simulink model "n99tot96reg55neu_10_8p"  (R2022b)
settings: Solver=VariableStepAuto  StartTime=0.0  StopTime=10.0  RelTol=1e-3
libraries: neural x61
(part 2 of 3)

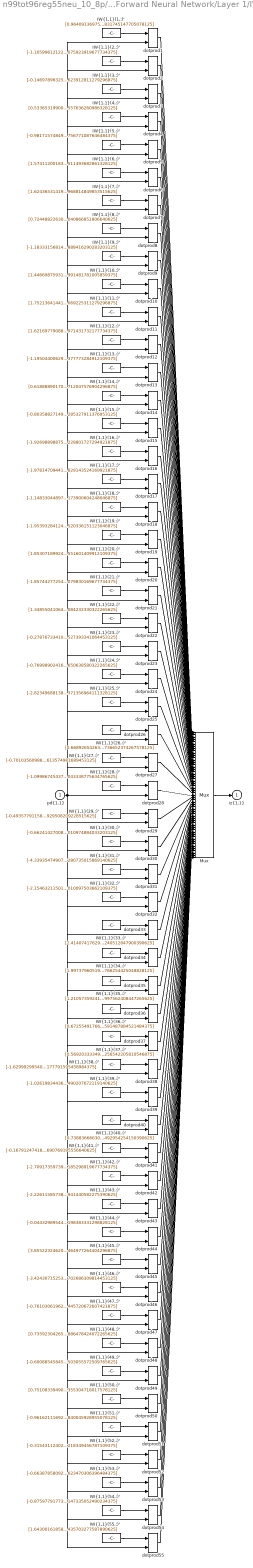
== system n99tot96reg55neu_10_8p/Feed-Forward Neural Network/Layer 1/IW{1,1} ==
  "pd{1,1}" : Inport  PortDimensions=7
      mask Display: e = 0.06;c1 = [120 230 180]/255;c2 = ([120 230 180]+0)/(256+128);c3 = ([120 230 180]+128)/(256+128);patch([0 1 1 0],[0 0 1 1],c1);patch([0 1 1 1-e 1-e 0+e],[0 0 1 1-e 0+e 0+e],c2);patch([0 0 1 1-e 0+e 0+e],[0 1 1 1-e 1-e 0+e],c3);plot([0 1 1 0 0],[0 0 1 1 0]);
  "IW{1,1}(1,:)'" : Constant  Value=[0.96409136975342180075898568247794173657894134521484375;-0.01177306743164707562854243150241018156521022319793701171875;1.5872895079200481927017563066328875720500946044921875;-0.67946510242392033074310120355221442878246307373046875;-1.3804786704522087337210223267902620136737823486328125;0.54905886044986174088222696809680201113224029541015625;0.1319087701998143125070583892011200077831745147705078125]
      mask Display: e = 0.06;c1 = [120 150 230]/255;c2 = ([120 150 230]+0)/383;c3 = ([120 150 230]+128)/383;patch([0 1 1 0],[0 0 1 1],c1);patch([0 1 1 1-e 1-e 0+e],[0 0 1 1-e 0+e 0+e],c2);patch([0 0 1 1-e 0+e 0+e],[0 1 1 1-e 1-e 0+e],c3);plot([0 1 1 0 0],[0 0 1 1 0]);disp('Weights');
  "IW{1,1}(10,:)'" : Constant  Value=[1.44669875931127744905779763939790427684783935546875;1.63028544792287721776347098057158291339874267578125;-0.402402933929877304475297705721459351480007171630859375;-1.5160626699661390315299058784148655831813812255859375;-0.59991510336130193792314457823522388935089111328125;4.485717304041894948340996052138507366180419921875;3.753049417834217305056654367945156991481781005859375]
      mask Display: e = 0.06;c1 = [120 150 230]/255;c2 = ([120 150 230]+0)/383;c3 = ([120 150 230]+128)/383;patch([0 1 1 0],[0 0 1 1],c1);patch([0 1 1 1-e 1-e 0+e],[0 0 1 1-e 0+e 0+e],c2);patch([0 0 1 1-e 0+e 0+e],[0 1 1 1-e 1-e 0+e],c3);plot([0 1 1 0 0],[0 0 1 1 0]);disp('Weights');
  "IW{1,1}(11,:)'" : Constant  Value=[1.7521364144150819441847488633356988430023193359375;0.374551279395318348353072224199422635138034820556640625;-0.8048865199683366000726891797967255115509033203125;-1.1542150106230366635173822942306287586688995361328125;-1.0925803363994777139822645040112547576427459716796875;3.507870265100738293995163985528051853179931640625;-0.35232665294651877019305175053887069225311279296875]
      mask Display: e = 0.06;c1 = [120 150 230]/255;c2 = ([120 150 230]+0)/383;c3 = ([120 150 230]+128)/383;patch([0 1 1 0],[0 0 1 1],c1);patch([0 1 1 1-e 1-e 0+e],[0 0 1 1-e 0+e 0+e],c2);patch([0 0 1 1-e 0+e 0+e],[0 1 1 1-e 1-e 0+e],c3);plot([0 1 1 0 0],[0 0 1 1 0]);disp('Weights');
  "IW{1,1}(12,:)'" : Constant  Value=[1.621697790883335432710055101779289543628692626953125;-1.027740414893572928889398099272511899471282958984375;0.52000990040676475789638288915739394724369049072265625;-1.2904215501701579160709343341295607388019561767578125;0.2070615557831251563047914032722474075853824615478515625;-0.62948300486669139797157868088106624782085418701171875;-0.148242942208577144214132204069755971431732177734375]
      mask Display: e = 0.06;c1 = [120 150 230]/255;c2 = ([120 150 230]+0)/383;c3 = ([120 150 230]+128)/383;patch([0 1 1 0],[0 0 1 1],c1);patch([0 1 1 1-e 1-e 0+e],[0 0 1 1-e 0+e 0+e],c2);patch([0 0 1 1-e 0+e 0+e],[0 1 1 1-e 1-e 0+e],c3);plot([0 1 1 0 0],[0 0 1 1 0]);disp('Weights');
  "IW{1,1}(13,:)'" : Constant  Value=[-1.1950440062912488503599206524086184799671173095703125;-0.2097753467574469954382010428162175230681896209716796875;-0.1785548924775699208833401598894852213561534881591796875;1.746302113315184367792198827373795211315155029296875;0.74511188216674117956728196077165193855762481689453125;-0.6065851337297212264587642494007013738155364990234375;0.69596479632327790110224441377795301377773284912109375]
      mask Display: e = 0.06;c1 = [120 150 230]/255;c2 = ([120 150 230]+0)/383;c3 = ([120 150 230]+128)/383;patch([0 1 1 0],[0 0 1 1],c1);patch([0 1 1 1-e 1-e 0+e],[0 0 1 1-e 0+e 0+e],c2);patch([0 0 1 1-e 0+e 0+e],[0 1 1 1-e 1-e 0+e],c3);plot([0 1 1 0 0],[0 0 1 1 0]);disp('Weights');
  "IW{1,1}(14,:)'" : Constant  Value=[0.61888890170968047232946673830156214535236358642578125;1.214752801341773658094780330429784953594207763671875;1.31303559531543356797556043602526187896728515625;2.5583165445786182345955239725299179553985595703125;0.1053019395176611194830940121391904540359973907470703125;-0.0849641386174930790531334423576481640338897705078125;-3.36967190537567073960190100478939712047576904296875]
      mask Display: e = 0.06;c1 = [120 150 230]/255;c2 = ([120 150 230]+0)/383;c3 = ([120 150 230]+128)/383;patch([0 1 1 0],[0 0 1 1],c1);patch([0 1 1 1-e 1-e 0+e],[0 0 1 1-e 0+e 0+e],c2);patch([0 0 1 1-e 0+e 0+e],[0 1 1 1-e 1-e 0+e],c3);plot([0 1 1 0 0],[0 0 1 1 0]);disp('Weights');
  "IW{1,1}(15,:)'" : Constant  Value=[-0.80358827149232492370600766662391833961009979248046875;0.498965545826864642631193191846250556409358978271484375;-0.8545972439642370854784303446649573743343353271484375;0.98441551894562329128035571557120420038700103759765625;0.12014292021084325978730333872590563260018825531005859375;-1.2101890103956451927302850890555419027805328369140625;-1.9228372444214134606710331354406662285327911376953125]
      mask Display: e = 0.06;c1 = [120 150 230]/255;c2 = ([120 150 230]+0)/383;c3 = ([120 150 230]+128)/383;patch([0 1 1 0],[0 0 1 1],c1);patch([0 1 1 1-e 1-e 0+e],[0 0 1 1-e 0+e 0+e],c2);patch([0 0 1 1-e 0+e 0+e],[0 1 1 1-e 1-e 0+e],c3);plot([0 1 1 0 0],[0 0 1 1 0]);disp('Weights');
  "IW{1,1}(16,:)'" : Constant  Value=[-1.9269889887593534272269835128099657595157623291015625;-0.2476305335269427254640817182007594965398311614990234375;2.488675633013846866248286460177041590213775634765625;-0.126684874263239433123118260482442565262317657470703125;-0.001767046437138157684298978011838698876090347766876220703125;-0.027095573409086463889661189341495628468692302703857421875;-4.03766240194085934689383066142909228801727294921875]
      mask Display: e = 0.06;c1 = [120 150 230]/255;c2 = ([120 150 230]+0)/383;c3 = ([120 150 230]+128)/383;patch([0 1 1 0],[0 0 1 1],c1);patch([0 1 1 1-e 1-e 0+e],[0 0 1 1-e 0+e 0+e],c2);patch([0 0 1 1-e 0+e 0+e],[0 1 1 1-e 1-e 0+e],c3);plot([0 1 1 0 0],[0 0 1 1 0]);disp('Weights');
  "IW{1,1}(17,:)'" : Constant  Value=[-1.9781470944136680945035777767770923674106597900390625;0.337505755853185263060112220045994035899639129638671875;0.9580014437199990684490558123798109591007232666015625;-0.28588062157459248613378122172434814274311065673828125;1.0385789812388448449809175144764594733715057373046875;-1.1184334967371227786969711814890615642070770263671875;0.45015646312713364363133905499125830829143524169921875]
      mask Display: e = 0.06;c1 = [120 150 230]/255;c2 = ([120 150 230]+0)/383;c3 = ([120 150 230]+128)/383;patch([0 1 1 0],[0 0 1 1],c1);patch([0 1 1 1-e 1-e 0+e],[0 0 1 1-e 0+e 0+e],c2);patch([0 0 1 1-e 0+e 0+e],[0 1 1 1-e 1-e 0+e],c3);plot([0 1 1 0 0],[0 0 1 1 0]);disp('Weights');
  "IW{1,1}(18,:)'" : Constant  Value=[-1.14833044897396963079927445505745708942413330078125;2.15389162668215394802473383606411516666412353515625;2.7733885104446915903508852352388203144073486328125;-1.626580994116236578150846980861388146877288818359375;-2.283818728665732322724579717032611370086669921875;-3.291976623125189238550092341029085218906402587890625;-8.0821552937094889301761213573627173900604248046875]
      mask Display: e = 0.06;c1 = [120 150 230]/255;c2 = ([120 150 230]+0)/383;c3 = ([120 150 230]+128)/383;patch([0 1 1 0],[0 0 1 1],c1);patch([0 1 1 1-e 1-e 0+e],[0 0 1 1-e 0+e 0+e],c2);patch([0 0 1 1-e 0+e 0+e],[0 1 1 1-e 1-e 0+e],c3);plot([0 1 1 0 0],[0 0 1 1 0]);disp('Weights');
  "IW{1,1}(19,:)'" : Constant  Value=[-1.9539328412408967228230949331191368401050567626953125;-2.217831340497449676973928944789804518222808837890625;-0.16820158276227292759585907333530485630035400390625;1.744154128670201142625728607526980340480804443359375;-0.861060806236878750752339328755624592304229736328125;-0.9103451453763022893639345056726597249507904052734375;-0.58368474434755224233839498992892913520336151123046875]
      mask Display: e = 0.06;c1 = [120 150 230]/255;c2 = ([120 150 230]+0)/383;c3 = ([120 150 230]+128)/383;patch([0 1 1 0],[0 0 1 1],c1);patch([0 1 1 1-e 1-e 0+e],[0 0 1 1-e 0+e 0+e],c2);patch([0 0 1 1-e 0+e 0+e],[0 1 1 1-e 1-e 0+e],c3);plot([0 1 1 0 0],[0 0 1 1 0]);disp('Weights');
  "IW{1,1}(2,:)'" : Constant  Value=[-1.10599612122139578929136405349709093570709228515625;1.680208229464801750197011642740108072757720947265625;-0.024762084197533777707445068472225102595984935760498046875;-0.425516864043877174328400769809377379715442657470703125;0.95366575580371548692681926695513539016246795654296875;-0.004666615684457037747934204929833867936395108699798583984375;2.030983216547548320107807739987038075923919677734375]
      mask Display: e = 0.06;c1 = [120 150 230]/255;c2 = ([120 150 230]+0)/383;c3 = ([120 150 230]+128)/383;patch([0 1 1 0],[0 0 1 1],c1);patch([0 1 1 1-e 1-e 0+e],[0 0 1 1-e 0+e 0+e],c2);patch([0 0 1 1-e 0+e 0+e],[0 1 1 1-e 1-e 0+e],c3);plot([0 1 1 0 0],[0 0 1 1 0]);disp('Weights');
  "IW{1,1}(20,:)'" : Constant  Value=[1.8530718992458978799930946479435078799724578857421875;2.2212717869272200488239832338877022266387939453125;1.876501287281657770478204838582314550876617431640625;-1.3501838911946111299045014675357379019260406494140625;-1.758042661725913280434951957431621849536895751953125;0.768034438087264792471842156373895704746246337890625;-1.829242199547669311954223303473554551601409912109375]
      mask Display: e = 0.06;c1 = [120 150 230]/255;c2 = ([120 150 230]+0)/383;c3 = ([120 150 230]+128)/383;patch([0 1 1 0],[0 0 1 1],c1);patch([0 1 1 1-e 1-e 0+e],[0 0 1 1-e 0+e 0+e],c2);patch([0 0 1 1-e 0+e 0+e],[0 1 1 1-e 1-e 0+e],c3);plot([0 1 1 0 0],[0 0 1 1 0]);disp('Weights');
  "IW{1,1}(21,:)'" : Constant  Value=[-1.8574427725451665427414127407246269285678863525390625;-0.41283790207952153483716983828344382345676422119140625;-0.334143875292905956353450847018393687903881072998046875;1.3382851087273535117816436468274332582950592041015625;2.874336028506728535347747310879640281200408935546875;-1.785792777279144871727112331427633762359619140625;0.2098256791471025672901618008836521767079830169677734375]
      mask Display: e = 0.06;c1 = [120 150 230]/255;c2 = ([120 150 230]+0)/383;c3 = ([120 150 230]+128)/383;patch([0 1 1 0],[0 0 1 1],c1);patch([0 1 1 1-e 1-e 0+e],[0 0 1 1-e 0+e 0+e],c2);patch([0 0 1 1-e 0+e 0+e],[0 1 1 1-e 1-e 0+e],c3);plot([0 1 1 0 0],[0 0 1 1 0]);disp('Weights');
  "IW{1,1}(22,:)'" : Constant  Value=[1.3485504106497689935650896586594171822071075439453125;1.2620957805625392378345850374898873269557952880859375;-0.3213557148957211229145514153060503304004669189453125;-3.395220299319527068604429587139748036861419677734375;0.231620104664224613078005177158047445118427276611328125;-0.78989915950265243704819795311777852475643157958984375;0.230443244263615787392751599327311851084232330322265625]
      mask Display: e = 0.06;c1 = [120 150 230]/255;c2 = ([120 150 230]+0)/383;c3 = ([120 150 230]+128)/383;patch([0 1 1 0],[0 0 1 1],c1);patch([0 1 1 1-e 1-e 0+e],[0 0 1 1-e 0+e 0+e],c2);patch([0 0 1 1-e 0+e 0+e],[0 1 1 1-e 1-e 0+e],c3);plot([0 1 1 0 0],[0 0 1 1 0]);disp('Weights');
  "IW{1,1}(23,:)'" : Constant  Value=[-0.27876733410687626335544564426527358591556549072265625;-0.10386558321394760706635196356728556565940380096435546875;-0.873790668035300921445696076261810958385467529296875;0.47768030623743651386092778921010904014110565185546875;1.36684305583762721880702883936464786529541015625;1.1757142426198192719510871029342524707317352294921875;-0.17711290702684767683905420199153013527393341064453125]
      mask Display: e = 0.06;c1 = [120 150 230]/255;c2 = ([120 150 230]+0)/383;c3 = ([120 150 230]+128)/383;patch([0 1 1 0],[0 0 1 1],c1);patch([0 1 1 1-e 1-e 0+e],[0 0 1 1-e 0+e 0+e],c2);patch([0 0 1 1-e 0+e 0+e],[0 1 1 1-e 1-e 0+e],c3);plot([0 1 1 0 0],[0 0 1 1 0]);disp('Weights');
  "IW{1,1}(24,:)'" : Constant  Value=[-0.76998902416556280758896946281311102211475372314453125;-2.044754804768209144327784088090993463993072509765625;-0.9332097446583886846127597891609184443950653076171875;0.64676073254784827160079885288723744451999664306640625;2.67022609839191016334325468051247298717498779296875;-1.8023100949980184193321974817081354558467864990234375;1.1399464868748572232703963891253806650638580322265625]
      mask Display: e = 0.06;c1 = [120 150 230]/255;c2 = ([120 150 230]+0)/383;c3 = ([120 150 230]+128)/383;patch([0 1 1 0],[0 0 1 1],c1);patch([0 1 1 1-e 1-e 0+e],[0 0 1 1-e 0+e 0+e],c2);patch([0 0 1 1-e 0+e 0+e],[0 1 1 1-e 1-e 0+e],c3);plot([0 1 1 0 0],[0 0 1 1 0]);disp('Weights');
  "IW{1,1}(25,:)'" : Constant  Value=[-2.82349688138738219578272037324495613574981689453125;-0.83664445390135278035614874170278199017047882080078125;0.032085039703056102144973493750512716360390186309814453125;1.234905292813121224781980345142073929309844970703125;-0.0387544861586598121672153638428426347672939300537109375;0.044237765068636185350481326850058394484221935272216796875;-1.916552761701712626063454081304371356964111328125]
      mask Display: e = 0.06;c1 = [120 150 230]/255;c2 = ([120 150 230]+0)/383;c3 = ([120 150 230]+128)/383;patch([0 1 1 0],[0 0 1 1],c1);patch([0 1 1 1-e 1-e 0+e],[0 0 1 1-e 0+e 0+e],c2);patch([0 0 1 1-e 0+e 0+e],[0 1 1 1-e 1-e 0+e],c3);plot([0 1 1 0 0],[0 0 1 1 0]);disp('Weights');
  "IW{1,1}(26,:)'" : Constant  Value=[0.668926542636925969276262549101375043392181396484375;1.8013448778058627208764619354042224586009979248046875;-1.1048519859487175853729468144592829048633575439453125;-1.38078111663339342385370400734245777130126953125;-0.2094143426941169339183801412218599580228328704833984375;0.64833955001450049859812452268670313060283660888671875;1.19004455055547442299257454578764736652374267578125]
      mask Display: e = 0.06;c1 = [120 150 230]/255;c2 = ([120 150 230]+0)/383;c3 = ([120 150 230]+128)/383;patch([0 1 1 0],[0 0 1 1],c1);patch([0 1 1 1-e 1-e 0+e],[0 0 1 1-e 0+e 0+e],c2);patch([0 0 1 1-e 0+e 0+e],[0 1 1 1-e 1-e 0+e],c3);plot([0 1 1 0 0],[0 0 1 1 0]);disp('Weights');
  "IW{1,1}(27,:)'" : Constant  Value=[-0.7010356098827428272812767318100668489933013916015625;-1.72879781811999233553933663642965257167816162109375;-1.211863422981742655082371129537932574748992919921875;-0.61965280025073654623923857798217795789241790771484375;2.379687656013285135259138769470155239105224609375;0.001000173054193870779415842520165824680589139461517333984375;-0.138460348853699788396198755435761995613574981689453125]
      mask Display: e = 0.06;c1 = [120 150 230]/255;c2 = ([120 150 230]+0)/383;c3 = ([120 150 230]+128)/383;patch([0 1 1 0],[0 0 1 1],c1);patch([0 1 1 1-e 1-e 0+e],[0 0 1 1-e 0+e 0+e],c2);patch([0 0 1 1-e 0+e 0+e],[0 1 1 1-e 1-e 0+e],c3);plot([0 1 1 0 0],[0 0 1 1 0]);disp('Weights');
  "IW{1,1}(28,:)'" : Constant  Value=[-1.099867454379433784339425983489491045475006103515625;-0.39164847347787679066044574938132427632808685302734375;0.2041264122213182208298576369998045265674591064453125;-1.3780747367931669433716024286695756018161773681640625;1.1160170869806698146220469425315968692302703857421875;2.39059811372251918015763294533826410770416259765625;-0.70933364882737370837872958873049356043338775634765625]
      mask Display: e = 0.06;c1 = [120 150 230]/255;c2 = ([120 150 230]+0)/383;c3 = ([120 150 230]+128)/383;patch([0 1 1 0],[0 0 1 1],c1);patch([0 1 1 1-e 1-e 0+e],[0 0 1 1-e 0+e 0+e],c2);patch([0 0 1 1-e 0+e 0+e],[0 1 1 1-e 1-e 0+e],c3);plot([0 1 1 0 0],[0 0 1 1 0]);disp('Weights');
  "IW{1,1}(29,:)'" : Constant  Value=[-0.49357791158585129220881526634912006556987762451171875;-1.058954600391138090031972751603461802005767822265625;0.6014563490360897990427702097804285585880279541015625;-2.3259698730596340965348645113408565521240234375;-0.9898491062698788756080148232285864651203155517578125;0.2027161471748838705853046349147916771471500396728515625;1.4431777195648383127490888000465929508209228515625]
      mask Display: e = 0.06;c1 = [120 150 230]/255;c2 = ([120 150 230]+0)/383;c3 = ([120 150 230]+128)/383;patch([0 1 1 0],[0 0 1 1],c1);patch([0 1 1 1-e 1-e 0+e],[0 0 1 1-e 0+e 0+e],c2);patch([0 0 1 1-e 0+e 0+e],[0 1 1 1-e 1-e 0+e],c3);plot([0 1 1 0 0],[0 0 1 1 0]);disp('Weights');
  "IW{1,1}(3,:)'" : Constant  Value=[-0.1469789632548356983487991556103224866092205047607421875;0.91802112737148988674817928767879493534564971923828125;-1.7315084354399810084856881076120771467685699462890625;2.2492375792367891307321770000271499156951904296875;-0.00930592123371699365963483074892792501486837863922119140625;-0.73742506180816735916749848911422304809093475341796875;0.75199550827603534042253841107594780623912811279296875]
      mask Display: e = 0.06;c1 = [120 150 230]/255;c2 = ([120 150 230]+0)/383;c3 = ([120 150 230]+128)/383;patch([0 1 1 0],[0 0 1 1],c1);patch([0 1 1 1-e 1-e 0+e],[0 0 1 1-e 0+e 0+e],c2);patch([0 0 1 1-e 0+e 0+e],[0 1 1 1-e 1-e 0+e],c3);plot([0 1 1 0 0],[0 0 1 1 0]);disp('Weights');
  "IW{1,1}(30,:)'" : Constant  Value=[-0.66241427008352038452443366622901521623134613037109375;0.328844704863163361796551953375455923378467559814453125;0.39030516842330342797140474431216716766357421875;3.480893476264444341694570539402775466442108154296875;-0.75690918307947419041425973773584701120853424072265625;0.83617571872394524934435366958496160805225372314453125;0.2851689363163547596968783182092010974884033203125]
      mask Display: e = 0.06;c1 = [120 150 230]/255;c2 = ([120 150 230]+0)/383;c3 = ([120 150 230]+128)/383;patch([0 1 1 0],[0 0 1 1],c1);patch([0 1 1 1-e 1-e 0+e],[0 0 1 1-e 0+e 0+e],c2);patch([0 0 1 1-e 0+e 0+e],[0 1 1 1-e 1-e 0+e],c3);plot([0 1 1 0 0],[0 0 1 1 0]);disp('Weights');
  "IW{1,1}(31,:)'" : Constant  Value=[-4.33935474907979834569005106459371745586395263671875;0.77532113981389871870675278842099942266941070556640625;-0.85932834286017090175135990648414008319377899169921875;-2.03451793702961492016356714884750545024871826171875;-0.58659820535468465418915684495004825294017791748046875;2.344161464210929413098938312032260000705718994140625;-2.14721443350844598541016239323653280735015869140625]
      mask Display: e = 0.06;c1 = [120 150 230]/255;c2 = ([120 150 230]+0)/383;c3 = ([120 150 230]+128)/383;patch([0 1 1 0],[0 0 1 1],c1);patch([0 1 1 1-e 1-e 0+e],[0 0 1 1-e 0+e 0+e],c2);patch([0 0 1 1-e 0+e 0+e],[0 1 1 1-e 1-e 0+e],c3);plot([0 1 1 0 0],[0 0 1 1 0]);disp('Weights');
  "IW{1,1}(32,:)'" : Constant  Value=[-2.154632115013669579894894923199899494647979736328125;2.52461796941434091223754876409657299518585205078125;2.7481629953011879052837684866972267627716064453125;-0.426651017390497211412281330922269262373447418212890625;1.4219593282147846569074545186595059931278228759765625;3.0614302866221922982958858483470976352691650390625;-1.7667034115813426975449829114950262010097503662109375]
      mask Display: e = 0.06;c1 = [120 150 230]/255;c2 = ([120 150 230]+0)/383;c3 = ([120 150 230]+128)/383;patch([0 1 1 0],[0 0 1 1],c1);patch([0 1 1 1-e 1-e 0+e],[0 0 1 1-e 0+e 0+e],c2);patch([0 0 1 1-e 0+e 0+e],[0 1 1 1-e 1-e 0+e],c3);plot([0 1 1 0 0],[0 0 1 1 0]);disp('Weights');
  "IW{1,1}(33,:)'" : Constant  Value=[2.41407417629160203631499825860373675823211669921875;-1.533856517398853203104636122588999569416046142578125;1.672630751004379856539117099600844085216522216796875;0.7826597390346179405895554737071506679058074951171875;-1.5988542944741686024912041830248199403285980224609375;-0.0358281874098995978261683603705023415386676788330078125;0.0239558467990849434381406268812497728504240512847900390625]
      mask Display: e = 0.06;c1 = [120 150 230]/255;c2 = ([120 150 230]+0)/383;c3 = ([120 150 230]+128)/383;patch([0 1 1 0],[0 0 1 1],c1);patch([0 1 1 1-e 1-e 0+e],[0 0 1 1-e 0+e 0+e],c2);patch([0 0 1 1-e 0+e 0+e],[0 1 1 1-e 1-e 0+e],c3);plot([0 1 1 0 0],[0 0 1 1 0]);disp('Weights');
  "IW{1,1}(34,:)'" : Constant  Value=[1.997379605196471619166231903363950550556182861328125;1.3289854560345173428714815599960274994373321533203125;1.60905575657723165505785800633020699024200439453125;0.398747680338293830626383851267746649682521820068359375;-0.0407896394768573478106787888464168645441532135009765625;0.296254961531278837583158747293055057525634765625;-0.701390170177618177405065580387599766254425048828125]
      mask Display: e = 0.06;c1 = [120 150 230]/255;c2 = ([120 150 230]+0)/383;c3 = ([120 150 230]+128)/383;patch([0 1 1 0],[0 0 1 1],c1);patch([0 1 1 1-e 1-e 0+e],[0 0 1 1-e 0+e 0+e],c2);patch([0 0 1 1-e 0+e 0+e],[0 1 1 1-e 1-e 0+e],c3);plot([0 1 1 0 0],[0 0 1 1 0]);disp('Weights');
  "IW{1,1}(35,:)'" : Constant  Value=[1.21057359241371553792987469932995736598968505859375;-0.8932981444597556386355563518009148538112640380859375;-1.877470439684020053761059898533858358860015869140625;0.7885600660692098085036150223459117114543914794921875;0.78624732612702386003178389728418551385402679443359375;2.191552339266968463249440901563502848148345947265625;3.340952984348723564522742890403605997562408447265625]
      mask Display: e = 0.06;c1 = [120 150 230]/255;c2 = ([120 150 230]+0)/383;c3 = ([120 150 230]+128)/383;patch([0 1 1 0],[0 0 1 1],c1);patch([0 1 1 1-e 1-e 0+e],[0 0 1 1-e 0+e 0+e],c2);patch([0 0 1 1-e 0+e 0+e],[0 1 1 1-e 1-e 0+e],c3);plot([0 1 1 0 0],[0 0 1 1 0]);disp('Weights');
  "IW{1,1}(36,:)'" : Constant  Value=[0.6725549176675063023367329151369631290435791015625;-1.306522824982356834055963190621696412563323974609375;1.9285415223230242265373135523987002670764923095703125;-0.168202127520857669384923838151735253632068634033203125;0.02775358505212451032395648553574574179947376251220703125;0.9260857311389740775808832040638662874698638916015625;-0.0670441685855417135453393484567641280591487884521484375]
      mask Display: e = 0.06;c1 = [120 150 230]/255;c2 = ([120 150 230]+0)/383;c3 = ([120 150 230]+128)/383;patch([0 1 1 0],[0 0 1 1],c1);patch([0 1 1 1-e 1-e 0+e],[0 0 1 1-e 0+e 0+e],c2);patch([0 0 1 1-e 0+e 0+e],[0 1 1 1-e 1-e 0+e],c3);plot([0 1 1 0 0],[0 0 1 1 0]);disp('Weights');
  "IW{1,1}(37,:)'" : Constant  Value=[0.56920333349400864531020260983495973050594329833984375;1.4545352963919999655928450010833330452442169189453125;0.50564817009018003801656959694810211658477783203125;1.0336611394723735912748452392406761646270751953125;0.85087876346725754839184219235903583467006683349609375;-0.562833581059996479467599783674813807010650634765625;-1.3281132140716731537821715392055921256542205810546875]
      mask Display: e = 0.06;c1 = [120 150 230]/255;c2 = ([120 150 230]+0)/383;c3 = ([120 150 230]+128)/383;patch([0 1 1 0],[0 0 1 1],c1);patch([0 1 1 1-e 1-e 0+e],[0 0 1 1-e 0+e 0+e],c2);patch([0 0 1 1-e 0+e 0+e],[0 1 1 1-e 1-e 0+e],c3);plot([0 1 1 0 0],[0 0 1 1 0]);disp('Weights');
  "IW{1,1}(38,:)'" : Constant  Value=[-1.629992995408185318950700093409977853298187255859375;0.9427086490016358677479502148344181478023529052734375;2.90003200728441346001318379421718418598175048828125;-1.994109265882975545736144340480677783489227294921875;-0.375794687484544642774864087186870165169239044189453125;0.8691438749864131008138201650581322610378265380859375;-5.8417755653080316591285736649297177791595458984375]
      mask Display: e = 0.06;c1 = [120 150 230]/255;c2 = ([120 150 230]+0)/383;c3 = ([120 150 230]+128)/383;patch([0 1 1 0],[0 0 1 1],c1);patch([0 1 1 1-e 1-e 0+e],[0 0 1 1-e 0+e 0+e],c2);patch([0 0 1 1-e 0+e 0+e],[0 1 1 1-e 1-e 0+e],c3);plot([0 1 1 0 0],[0 0 1 1 0]);disp('Weights');
  "IW{1,1}(39,:)'" : Constant  Value=[-1.026198344360594649771201147814281284809112548828125;1.714101036310324843725538812577724456787109375;0.98260685412509818359438895640778355300426483154296875;-0.49267511848511380545545534914708696305751800537109375;2.021100531018337864708200868335552513599395751953125;0.383204925363066661869737572487792931497097015380859375;0.8095870562047695617735598716535605490207672119140625]
      mask Display: e = 0.06;c1 = [120 150 230]/255;c2 = ([120 150 230]+0)/383;c3 = ([120 150 230]+128)/383;patch([0 1 1 0],[0 0 1 1],c1);patch([0 1 1 1-e 1-e 0+e],[0 0 1 1-e 0+e 0+e],c2);patch([0 0 1 1-e 0+e 0+e],[0 1 1 1-e 1-e 0+e],c3);plot([0 1 1 0 0],[0 0 1 1 0]);disp('Weights');
  "IW{1,1}(4,:)'" : Constant  Value=[0.5336531990025321636750277320970781147480010986328125;0.201008486413918052715388284923392347991466522216796875;1.78743638430836426778114400804042816162109375;-1.771308146456824328396351120318286120891571044921875;-2.365201553805913459171961221727542579174041748046875;0.08585498338459231215669120729216956533491611480712890625;-0.90739037972411040744447063843836076557636260986328125]
      mask Display: e = 0.06;c1 = [120 150 230]/255;c2 = ([120 150 230]+0)/383;c3 = ([120 150 230]+128)/383;patch([0 1 1 0],[0 0 1 1],c1);patch([0 1 1 1-e 1-e 0+e],[0 0 1 1-e 0+e 0+e],c2);patch([0 0 1 1-e 0+e 0+e],[0 1 1 1-e 1-e 0+e],c3);plot([0 1 1 0 0],[0 0 1 1 0]);disp('Weights');
  "IW{1,1}(40,:)'" : Constant  Value=[0.73883666630786237750072587004979141056537628173828125;0.64093930136925703067163340165279805660247802734375;-1.5806062221313557092372548140701837837696075439453125;0.47340482841353537235562498608487658202648162841796875;1.727127563094725370973492317716591060161590576171875;0.976714277484310056109961806214414536952972412109375;1.543395893951976294289352154009975492954254150390625]
      mask Display: e = 0.06;c1 = [120 150 230]/255;c2 = ([120 150 230]+0)/383;c3 = ([120 150 230]+128)/383;patch([0 1 1 0],[0 0 1 1],c1);patch([0 1 1 1-e 1-e 0+e],[0 0 1 1-e 0+e 0+e],c2);patch([0 0 1 1-e 0+e 0+e],[0 1 1 1-e 1-e 0+e],c3);plot([0 1 1 0 0],[0 0 1 1 0]);disp('Weights');
  "IW{1,1}(41,:)'" : Constant  Value=[-0.1679124741854139124530576054894481785595417022705078125;-2.01412411911410327292060173931531608104705810546875;-1.0623156942214146969405419440590776503086090087890625;-2.290076869178389262771133871865458786487579345703125;-0.354599067359675224064829990311409346759319305419921875;-0.96817841007497185135122208521352149546146392822265625;-1.0633082790039767306922158240922726690769195556640625]
      mask Display: e = 0.06;c1 = [120 150 230]/255;c2 = ([120 150 230]+0)/383;c3 = ([120 150 230]+128)/383;patch([0 1 1 0],[0 0 1 1],c1);patch([0 1 1 1-e 1-e 0+e],[0 0 1 1-e 0+e 0+e],c2);patch([0 0 1 1-e 0+e 0+e],[0 1 1 1-e 1-e 0+e],c3);plot([0 1 1 0 0],[0 0 1 1 0]);disp('Weights');
  "IW{1,1}(42,:)'" : Constant  Value=[-2.709173597398663702051635482348501682281494140625;1.6923092883532009356173375635989941656589508056640625;0.95634613859526884649397970861173234879970550537109375;0.400215977678154033458923777288873679935932159423828125;0.7070198576079926855442181476973928511142730712890625;0.5382245516218404635111483003129251301288604736328125;1.724116162049477818385412319912575185298919677734375]
      mask Display: e = 0.06;c1 = [120 150 230]/255;c2 = ([120 150 230]+0)/383;c3 = ([120 150 230]+128)/383;patch([0 1 1 0],[0 0 1 1],c1);patch([0 1 1 1-e 1-e 0+e],[0 0 1 1-e 0+e 0+e],c2);patch([0 0 1 1-e 0+e 0+e],[0 1 1 1-e 1-e 0+e],c3);plot([0 1 1 0 0],[0 0 1 1 0]);disp('Weights');
  "IW{1,1}(43,:)'" : Constant  Value=[-2.226115857383809792935380755807273089885711669921875;0.93987453685519717350160817659343592822551727294921875;-0.30375794090971497407593915340839885175228118896484375;-0.713649215232978750833581216284073889255523681640625;0.2206496803574848619700077279048855416476726531982421875;1.91550047363819775370075149112381041049957275390625;1.579952698501268404385200483375228941440582275390625]
      mask Display: e = 0.06;c1 = [120 150 230]/255;c2 = ([120 150 230]+0)/383;c3 = ([120 150 230]+128)/383;patch([0 1 1 0],[0 0 1 1],c1);patch([0 1 1 1-e 1-e 0+e],[0 0 1 1-e 0+e 0+e],c2);patch([0 0 1 1-e 0+e 0+e],[0 1 1 1-e 1-e 0+e],c3);plot([0 1 1 0 0],[0 0 1 1 0]);disp('Weights');
  "IW{1,1}(44,:)'" : Constant  Value=[-0.044329895443299550950033705021269270218908786773681640625;1.13763376208977629033824996440671384334564208984375;-0.19374810487895766097921068649156950414180755615234375;1.9488956309318845594447111579938791692256927490234375;-1.8155061547943638355917528315330855548381805419921875;0.61883726032954522455753476606332696974277496337890625;-0.1524224364841990919661185444056172855198383331298828125]
      mask Display: e = 0.06;c1 = [120 150 230]/255;c2 = ([120 150 230]+0)/383;c3 = ([120 150 230]+128)/383;patch([0 1 1 0],[0 0 1 1],c1);patch([0 1 1 1-e 1-e 0+e],[0 0 1 1-e 0+e 0+e],c2);patch([0 0 1 1-e 0+e 0+e],[0 1 1 1-e 1-e 0+e],c3);plot([0 1 1 0 0],[0 0 1 1 0]);disp('Weights');
  "IW{1,1}(45,:)'" : Constant  Value=[3.855223246202371445434664565254934132099151611328125;-5.14310875034772951863715206854976713657379150390625;-1.668481689055025807277843341580592095851898193359375;0.375277734102789917169928912699106149375438690185546875;2.220726568371177211957956387777812778949737548828125;-0.97215901807749804941494176091509871184825897216796875;-0.77767470035851982146368754911236464977264404296875]
      mask Display: e = 0.06;c1 = [120 150 230]/255;c2 = ([120 150 230]+0)/383;c3 = ([120 150 230]+128)/383;patch([0 1 1 0],[0 0 1 1],c1);patch([0 1 1 1-e 1-e 0+e],[0 0 1 1-e 0+e 0+e],c2);patch([0 0 1 1-e 0+e 0+e],[0 1 1 1-e 1-e 0+e],c3);plot([0 1 1 0 0],[0 0 1 1 0]);disp('Weights');
  "IW{1,1}(46,:)'" : Constant  Value=[-3.42430715253043249646225376636721193790435791015625;-0.04391400767853481656999292681575752794742584228515625;-0.80989506088073170975150105732609517872333526611328125;-0.45439127770815124218728442428982816636562347412109375;1.33497189864738086129136718227528035640716552734375;1.8503960771579812671916442923247814178466796875;-1.1134401622587166702516014993307180702686309814453125]
      mask Display: e = 0.06;c1 = [120 150 230]/255;c2 = ([120 150 230]+0)/383;c3 = ([120 150 230]+128)/383;patch([0 1 1 0],[0 0 1 1],c1);patch([0 1 1 1-e 1-e 0+e],[0 0 1 1-e 0+e 0+e],c2);patch([0 0 1 1-e 0+e 0+e],[0 1 1 1-e 1-e 0+e],c3);plot([0 1 1 0 0],[0 0 1 1 0]);disp('Weights');
  "IW{1,1}(47,:)'" : Constant  Value=[-0.76103061962891371816652963389060460031032562255859375;-0.6474148229473986049242739682085812091827392578125;0.970739001414433033687600982375442981719970703125;-1.2605799641703721025720597026520408689975738525390625;0.38834820787214052728586466400884091854095458984375;0.54140476875808507539744596215314231812953948974609375;-2.7754526160805426115985028445720672607421875]
      mask Display: e = 0.06;c1 = [120 150 230]/255;c2 = ([120 150 230]+0)/383;c3 = ([120 150 230]+128)/383;patch([0 1 1 0],[0 0 1 1],c1);patch([0 1 1 1-e 1-e 0+e],[0 0 1 1-e 0+e 0+e],c2);patch([0 0 1 1-e 0+e 0+e],[0 1 1 1-e 1-e 0+e],c3);plot([0 1 1 0 0],[0 0 1 1 0]);disp('Weights');
  "IW{1,1}(48,:)'" : Constant  Value=[0.73592304265450370071022234697011299431324005126953125;-0.47887272950795456427641738628153689205646514892578125;-1.107777667627034556829812572686932981014251708984375;1.7676956183234338038090527334134094417095184326171875;1.7879629287546094928984530270099639892578125;-0.98089853793980597007617916460731066763401031494140625;3.361831801784779916175693870172835886478424072265625]
      mask Display: e = 0.06;c1 = [120 150 230]/255;c2 = ([120 150 230]+0)/383;c3 = ([120 150 230]+128)/383;patch([0 1 1 0],[0 0 1 1],c1);patch([0 1 1 1-e 1-e 0+e],[0 0 1 1-e 0+e 0+e],c2);patch([0 0 1 1-e 0+e 0+e],[0 1 1 1-e 1-e 0+e],c3);plot([0 1 1 0 0],[0 0 1 1 0]);disp('Weights');
  "IW{1,1}(49,:)'" : Constant  Value=[-0.60088545845568852588058916808222420513629913330078125;-0.64728852062445663140266560731106437742710113525390625;-1.173644541501836169317130043054930865764617919921875;-4.99896620028586458062136443913914263248443603515625;0.986208490362581624566473692539148032665252685546875;0.09938236786870956185335757027132785879075527191162109375;-1.0379858057904576273955399301485158503055572509765625]
      mask Display: e = 0.06;c1 = [120 150 230]/255;c2 = ([120 150 230]+0)/383;c3 = ([120 150 230]+128)/383;patch([0 1 1 0],[0 0 1 1],c1);patch([0 1 1 1-e 1-e 0+e],[0 0 1 1-e 0+e 0+e],c2);patch([0 0 1 1-e 0+e 0+e],[0 1 1 1-e 1-e 0+e],c3);plot([0 1 1 0 0],[0 0 1 1 0]);disp('Weights');
  "IW{1,1}(5,:)'" : Constant  Value=[-0.9817157484976937187326484490768052637577056884765625;-0.415149103162948229783779652279918082058429718017578125;-0.59731630424003245849462473415769636631011962890625;0.60195482486667462040941245504654943943023681640625;0.302771120356097156456343100217054598033428192138671875;2.768180076356405283632966529694385826587677001953125;-0.74512044826162637800592847270308993756771087646484375]
      mask Display: e = 0.06;c1 = [120 150 230]/255;c2 = ([120 150 230]+0)/383;c3 = ([120 150 230]+128)/383;patch([0 1 1 0],[0 0 1 1],c1);patch([0 1 1 1-e 1-e 0+e],[0 0 1 1-e 0+e 0+e],c2);patch([0 0 1 1-e 0+e 0+e],[0 1 1 1-e 1-e 0+e],c3);plot([0 1 1 0 0],[0 0 1 1 0]);disp('Weights');
  "IW{1,1}(50,:)'" : Constant  Value=[0.75108339490590891873722512173117138445377349853515625;0.1858762782421672365984477437450550496578216552734375;0.50504895915728387212340066980686970055103302001953125;0.19645766694630228954565609456039965152740478515625;-0.1662605427574199434825885646205279044806957244873046875;-1.86425545444731621813616584404371678829193115234375;1.5532481410189848958225411479361355304718017578125]
      mask Display: e = 0.06;c1 = [120 150 230]/255;c2 = ([120 150 230]+0)/383;c3 = ([120 150 230]+128)/383;patch([0 1 1 0],[0 0 1 1],c1);patch([0 1 1 1-e 1-e 0+e],[0 0 1 1-e 0+e 0+e],c2);patch([0 0 1 1-e 0+e 0+e],[0 1 1 1-e 1-e 0+e],c3);plot([0 1 1 0 0],[0 0 1 1 0]);disp('Weights');
  "IW{1,1}(51,:)'" : Constant  Value=[-0.96162111692733975853997208105283789336681365966796875;-2.2077083514502806593782224808819591999053955078125;-1.8742821840517265297165749871055595576763153076171875;2.203469933700599181491952549549750983715057373046875;-0.302347480317674166538921554092667065560817718505859375;0.640282629377079803845163041842170059680938720703125;1.8030254766071600602828084447537548840045928955078125]
      mask Display: e = 0.06;c1 = [120 150 230]/255;c2 = ([120 150 230]+0)/383;c3 = ([120 150 230]+128)/383;patch([0 1 1 0],[0 0 1 1],c1);patch([0 1 1 1-e 1-e 0+e],[0 0 1 1-e 0+e 0+e],c2);patch([0 0 1 1-e 0+e 0+e],[0 1 1 1-e 1-e 0+e],c3);plot([0 1 1 0 0],[0 0 1 1 0]);disp('Weights');
  "IW{1,1}(52,:)'" : Constant  Value=[-0.315431124027934772779957484090118668973445892333984375;0.6694608859951973744983888536808080971240997314453125;0.2455298404817331803240421095324563793838024139404296875;1.503832857747334106335301839862950146198272705078125;0.3871840962687134179986969684250652790069580078125;3.02975640550594871314160627662204205989837646484375;-0.53366024408075352081226583322859369218349456787109375]
      mask Display: e = 0.06;c1 = [120 150 230]/255;c2 = ([120 150 230]+0)/383;c3 = ([120 150 230]+128)/383;patch([0 1 1 0],[0 0 1 1],c1);patch([0 1 1 1-e 1-e 0+e],[0 0 1 1-e 0+e 0+e],c2);patch([0 0 1 1-e 0+e 0+e],[0 1 1 1-e 1-e 0+e],c3);plot([0 1 1 0 0],[0 0 1 1 0]);disp('Weights');
  "IW{1,1}(53,:)'" : Constant  Value=[-0.6638785809201237508858639557729475200176239013671875;0.98778733568180954183191033735056407749652862548828125;1.5520553206222105213640816145925782620906829833984375;-1.06672553812642245674169316771440207958221435546875;0.405924217941061871162133911639102734625339508056640625;-0.79541483981623439802888242411427199840545654296875;-0.570381780302839924701174822985194623470306396484375]
      mask Display: e = 0.06;c1 = [120 150 230]/255;c2 = ([120 150 230]+0)/383;c3 = ([120 150 230]+128)/383;patch([0 1 1 0],[0 0 1 1],c1);patch([0 1 1 1-e 1-e 0+e],[0 0 1 1-e 0+e 0+e],c2);patch([0 0 1 1-e 0+e 0+e],[0 1 1 1-e 1-e 0+e],c3);plot([0 1 1 0 0],[0 0 1 1 0]);disp('Weights');
  "IW{1,1}(54,:)'" : Constant  Value=[-0.87597791773202260401376406662166118621826171875;1.07209860140361268321385068702511489391326904296875;-1.32089558962827791077643269090913236141204833984375;0.471026188176155546916135108403977937996387481689453125;1.130144554373659904200621895142830908298492431640625;1.3178311248573433278608035834622569382190704345703125;-1.3511498560306571814493281635805033147335052490234375]
      mask Display: e = 0.06;c1 = [120 150 230]/255;c2 = ([120 150 230]+0)/383;c3 = ([120 150 230]+128)/383;patch([0 1 1 0],[0 0 1 1],c1);patch([0 1 1 1-e 1-e 0+e],[0 0 1 1-e 0+e 0+e],c2);patch([0 0 1 1-e 0+e 0+e],[0 1 1 1-e 1-e 0+e],c3);plot([0 1 1 0 0],[0 0 1 1 0]);disp('Weights');
  "IW{1,1}(55,:)'" : Constant  Value=[1.6430016185847293730404317102511413395404815673828125;0.23331223399436218368663276123697869479656219482421875;0.1916448081390855484595903135414118878543376922607421875;1.6883391862576597741707473687711171805858612060546875;-0.48729396450212847380356606663553975522518157958984375;1.222355186200739129986914122127927839756011962890625;-0.81712656991699683661778408350073732435703277587890625]
      mask Display: e = 0.06;c1 = [120 150 230]/255;c2 = ([120 150 230]+0)/383;c3 = ([120 150 230]+128)/383;patch([0 1 1 0],[0 0 1 1],c1);patch([0 1 1 1-e 1-e 0+e],[0 0 1 1-e 0+e 0+e],c2);patch([0 0 1 1-e 0+e 0+e],[0 1 1 1-e 1-e 0+e],c3);plot([0 1 1 0 0],[0 0 1 1 0]);disp('Weights');
  "IW{1,1}(6,:)'" : Constant  Value=[1.5741120018348710996036743381409905850887298583984375;-0.146234130279785989880991792233544401824474334716796875;1.4108745409749590127290730379172600805759429931640625;-0.0829913986708263606839608428344945423305034637451171875;-1.38716015198710262978920582099817693233489990234375;0.56871118229575345903725747120915912091732025146484375;0.53141573015021237313959545645047910511493682861328125]
      mask Display: e = 0.06;c1 = [120 150 230]/255;c2 = ([120 150 230]+0)/383;c3 = ([120 150 230]+128)/383;patch([0 1 1 0],[0 0 1 1],c1);patch([0 1 1 1-e 1-e 0+e],[0 0 1 1-e 0+e 0+e],c2);patch([0 0 1 1-e 0+e 0+e],[0 1 1 1-e 1-e 0+e],c3);plot([0 1 1 0 0],[0 0 1 1 0]);disp('Weights');
  "IW{1,1}(7,:)'" : Constant  Value=[1.624365314197401044538082715007476508617401123046875;-1.550490793845559434060987769044004380702972412109375;1.0626299838374697603882168550626374781131744384765625;-0.83385649425622687669346078109811060130596160888671875;0.5076710185933119845458350027911365032196044921875;0.278642275821545049030447671611909754574298858642578125;0.5734646328516659341545391725958324968814849853515625]
      mask Display: e = 0.06;c1 = [120 150 230]/255;c2 = ([120 150 230]+0)/383;c3 = ([120 150 230]+128)/383;patch([0 1 1 0],[0 0 1 1],c1);patch([0 1 1 1-e 1-e 0+e],[0 0 1 1-e 0+e 0+e],c2);patch([0 0 1 1-e 0+e 0+e],[0 1 1 1-e 1-e 0+e],c3);plot([0 1 1 0 0],[0 0 1 1 0]);disp('Weights');
  "IW{1,1}(8,:)'" : Constant  Value=[0.72448822630726483762231282526045106351375579833984375;-1.058180359926959024363668504520319402217864990234375;0.68939312128649576916217256439267657697200775146484375;-0.72025882160856713465335587898152880370616912841796875;-0.2318912990754060932108160386633244343101978302001953125;1.5502576756917647582412200790713541209697723388671875;0.60783474549953242505040407195338048040866851806640625]
      mask Display: e = 0.06;c1 = [120 150 230]/255;c2 = ([120 150 230]+0)/383;c3 = ([120 150 230]+128)/383;patch([0 1 1 0],[0 0 1 1],c1);patch([0 1 1 1-e 1-e 0+e],[0 0 1 1-e 0+e 0+e],c2);patch([0 0 1 1-e 0+e 0+e],[0 1 1 1-e 1-e 0+e],c3);plot([0 1 1 0 0],[0 0 1 1 0]);disp('Weights');
  "IW{1,1}(9,:)'" : Constant  Value=[-1.1833315681477529768272916044224984943866729736328125;-1.398909269830311163929081885726191103458404541015625;-1.6600215897117180929853930138051509857177734375;-6.59412026678810381241646609851159155368804931640625;3.9931196267699089474945139954797923564910888671875;0.2550501983339608091938544021104462444782257080078125;-0.72730108522929282077740253953379578888416290283203125]
      mask Display: e = 0.06;c1 = [120 150 230]/255;c2 = ([120 150 230]+0)/383;c3 = ([120 150 230]+128)/383;patch([0 1 1 0],[0 0 1 1],c1);patch([0 1 1 1-e 1-e 0+e],[0 0 1 1-e 0+e 0+e],c2);patch([0 0 1 1-e 0+e 0+e],[0 1 1 1-e 1-e 0+e],c3);plot([0 1 1 0 0],[0 0 1 1 0]);disp('Weights');
  Mux : Mux  Inputs=55
      mask Display: e = 0.06;c1 = [120 150 230]/255;c2 = ([120 150 230]+0)/383;c3 = ([120 150 230]+128)/383;patch([0 1 1 0],[0 0 1 1],c1);patch([0 1 1 1-e 1-e 0+e],[0 0 1 1-e 0+e 0+e],c2);patch([0 0 1 1-e 0+e 0+e],[0 1 1 1-e 1-e 0+e],c3);plot([0 1 1 0 0],[0 0 1 1 0]);disp('Mux');
  dotprod{1..55} (55 alike) : neural/Weight Functions/dotprod
  "iz{1,1}" : Outport
      mask Display: e = 0.06;c1 = [120 230 180]/255;c2 = ([120 230 180]+0)/(256+128);c3 = ([120 230 180]+128)/(256+128);patch([0 1 1 0],[0 0 1 1],c1);patch([0 1 1 1-e 1-e 0+e],[0 0 1 1-e 0+e 0+e],c2);patch([0 0 1 1-e 0+e 0+e],[0 1 1 1-e 1-e 0+e],c3);plot([0 1 1 0 0],[0 0 1 1 0]);
  wires:
  "IW{1,1}(1,:)'"/1 -> dotprod1/1
  "pd{1,1}"/1 -> dotprod1/2, dotprod2/2, dotprod3/2, dotprod4/2, dotprod5/2, dotprod6/2, dotprod7/2, dotprod8/2, dotprod9/2, dotprod10/2, dotprod11/2, dotprod12/2, dotprod13/2, dotprod14/2, dotprod15/2, dotprod16/2, dotprod17/2, dotprod18/2, dotprod19/2, dotprod20/2, dotprod21/2, dotprod22/2, dotprod23/2, dotprod24/2, dotprod25/2, dotprod26/2, dotprod27/2, dotprod28/2, dotprod29/2, dotprod30/2, dotprod31/2, dotprod32/2, dotprod33/2, dotprod34/2, dotprod35/2, dotprod36/2, dotprod37/2, dotprod38/2, dotprod39/2, dotprod40/2, dotprod41/2, dotprod42/2, dotprod43/2, dotprod44/2, dotprod45/2, dotprod46/2, dotprod47/2, dotprod48/2, dotprod49/2, dotprod50/2, dotprod51/2, dotprod52/2, dotprod53/2, dotprod54/2, dotprod55/2
  dotprod1/1 -> Mux/1
  "IW{1,1}(2,:)'"/1 -> dotprod2/1
  dotprod2/1 -> Mux/2
  "IW{1,1}(3,:)'"/1 -> dotprod3/1
  dotprod3/1 -> Mux/3
  "IW{1,1}(4,:)'"/1 -> dotprod4/1
  dotprod4/1 -> Mux/4
  "IW{1,1}(5,:)'"/1 -> dotprod5/1
  dotprod5/1 -> Mux/5
  "IW{1,1}(6,:)'"/1 -> dotprod6/1
  dotprod6/1 -> Mux/6
  "IW{1,1}(7,:)'"/1 -> dotprod7/1
  dotprod7/1 -> Mux/7
  "IW{1,1}(8,:)'"/1 -> dotprod8/1
  dotprod8/1 -> Mux/8
  "IW{1,1}(9,:)'"/1 -> dotprod9/1
  dotprod9/1 -> Mux/9
  "IW{1,1}(10,:)'"/1 -> dotprod10/1
  dotprod10/1 -> Mux/10
  "IW{1,1}(11,:)'"/1 -> dotprod11/1
  dotprod11/1 -> Mux/11
  "IW{1,1}(12,:)'"/1 -> dotprod12/1
  dotprod12/1 -> Mux/12
  "IW{1,1}(13,:)'"/1 -> dotprod13/1
  dotprod13/1 -> Mux/13
  "IW{1,1}(14,:)'"/1 -> dotprod14/1
  dotprod14/1 -> Mux/14
  "IW{1,1}(15,:)'"/1 -> dotprod15/1
  dotprod15/1 -> Mux/15
  "IW{1,1}(16,:)'"/1 -> dotprod16/1
  dotprod16/1 -> Mux/16
  "IW{1,1}(17,:)'"/1 -> dotprod17/1
  dotprod17/1 -> Mux/17
  "IW{1,1}(18,:)'"/1 -> dotprod18/1
  dotprod18/1 -> Mux/18
  "IW{1,1}(19,:)'"/1 -> dotprod19/1
  dotprod19/1 -> Mux/19
  "IW{1,1}(20,:)'"/1 -> dotprod20/1
  dotprod20/1 -> Mux/20
  "IW{1,1}(21,:)'"/1 -> dotprod21/1
  dotprod21/1 -> Mux/21
  "IW{1,1}(22,:)'"/1 -> dotprod22/1
  dotprod22/1 -> Mux/22
  "IW{1,1}(23,:)'"/1 -> dotprod23/1
  dotprod23/1 -> Mux/23
  "IW{1,1}(24,:)'"/1 -> dotprod24/1
  dotprod24/1 -> Mux/24
  "IW{1,1}(25,:)'"/1 -> dotprod25/1
  dotprod25/1 -> Mux/25
  "IW{1,1}(26,:)'"/1 -> dotprod26/1
  dotprod26/1 -> Mux/26
  "IW{1,1}(27,:)'"/1 -> dotprod27/1
  dotprod27/1 -> Mux/27
  "IW{1,1}(28,:)'"/1 -> dotprod28/1
  dotprod28/1 -> Mux/28
  "IW{1,1}(29,:)'"/1 -> dotprod29/1
  dotprod29/1 -> Mux/29
  "IW{1,1}(30,:)'"/1 -> dotprod30/1
  dotprod30/1 -> Mux/30
  "IW{1,1}(31,:)'"/1 -> dotprod31/1
  dotprod31/1 -> Mux/31
  "IW{1,1}(32,:)'"/1 -> dotprod32/1
  dotprod32/1 -> Mux/32
  "IW{1,1}(33,:)'"/1 -> dotprod33/1
  dotprod33/1 -> Mux/33
  "IW{1,1}(34,:)'"/1 -> dotprod34/1
  dotprod34/1 -> Mux/34
  "IW{1,1}(35,:)'"/1 -> dotprod35/1
  dotprod35/1 -> Mux/35
  "IW{1,1}(36,:)'"/1 -> dotprod36/1
  dotprod36/1 -> Mux/36
  "IW{1,1}(37,:)'"/1 -> dotprod37/1
  dotprod37/1 -> Mux/37
  "IW{1,1}(38,:)'"/1 -> dotprod38/1
  dotprod38/1 -> Mux/38
  "IW{1,1}(39,:)'"/1 -> dotprod39/1
  dotprod39/1 -> Mux/39
  "IW{1,1}(40,:)'"/1 -> dotprod40/1
  dotprod40/1 -> Mux/40
  "IW{1,1}(41,:)'"/1 -> dotprod41/1
  dotprod41/1 -> Mux/41
  "IW{1,1}(42,:)'"/1 -> dotprod42/1
  dotprod42/1 -> Mux/42
  "IW{1,1}(43,:)'"/1 -> dotprod43/1
  dotprod43/1 -> Mux/43
  "IW{1,1}(44,:)'"/1 -> dotprod44/1
  dotprod44/1 -> Mux/44
  "IW{1,1}(45,:)'"/1 -> dotprod45/1
  dotprod45/1 -> Mux/45
  "IW{1,1}(46,:)'"/1 -> dotprod46/1
  dotprod46/1 -> Mux/46
  "IW{1,1}(47,:)'"/1 -> dotprod47/1
  dotprod47/1 -> Mux/47
  "IW{1,1}(48,:)'"/1 -> dotprod48/1
  dotprod48/1 -> Mux/48
  "IW{1,1}(49,:)'"/1 -> dotprod49/1
  dotprod49/1 -> Mux/49
  "IW{1,1}(50,:)'"/1 -> dotprod50/1
  dotprod50/1 -> Mux/50
  "IW{1,1}(51,:)'"/1 -> dotprod51/1
  dotprod51/1 -> Mux/51
  "IW{1,1}(52,:)'"/1 -> dotprod52/1
  dotprod52/1 -> Mux/52
  "IW{1,1}(53,:)'"/1 -> dotprod53/1
  dotprod53/1 -> Mux/53
  "IW{1,1}(54,:)'"/1 -> dotprod54/1
  dotprod54/1 -> Mux/54
  "IW{1,1}(55,:)'"/1 -> dotprod55/1
  dotprod55/1 -> Mux/55
  Mux/1 -> "iz{1,1}"/1

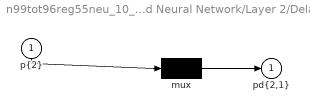
== system n99tot96reg55neu_10_8p/Feed-Forward Neural Network/Layer 2/Delays 1 ==
  "p{2}" : Inport  PortDimensions=55
      mask Display: e = 0.06;c1 = [120 230 180]/255;c2 = ([120 230 180]+0)/(256+128);c3 = ([120 230 180]+128)/(256+128);patch([0 1 1 0],[0 0 1 1],c1);patch([0 1 1 1-e 1-e 0+e],[0 0 1 1-e 0+e 0+e],c2);patch([0 0 1 1-e 0+e 0+e],[0 1 1 1-e 1-e 0+e],c3);plot([0 1 1 0 0],[0 0 1 1 0]);
  mux : Mux  Inputs=1
      mask Display: e = 0.06;c1 = [120 150 230]/255;c2 = ([120 150 230]+0)/383;c3 = ([120 150 230]+128)/383;patch([0 1 1 0],[0 0 1 1],c1);patch([0 1 1 1-e 1-e 0+e],[0 0 1 1-e 0+e 0+e],c2);patch([0 0 1 1-e 0+e 0+e],[0 1 1 1-e 1-e 0+e],c3);plot([0 1 1 0 0],[0 0 1 1 0]);disp('Mux')
  "pd{2,1}" : Outport
      mask Display: e = 0.06;c1 = [120 230 180]/255;c2 = ([120 230 180]+0)/(256+128);c3 = ([120 230 180]+128)/(256+128);patch([0 1 1 0],[0 0 1 1],c1);patch([0 1 1 1-e 1-e 0+e],[0 0 1 1-e 0+e 0+e],c2);patch([0 0 1 1-e 0+e 0+e],[0 1 1 1-e 1-e 0+e],c3);plot([0 1 1 0 0],[0 0 1 1 0]);
  wires:
  "p{2}"/1 -> mux/1
  mux/1 -> "pd{2,1}"/1
